simulink model "D53_LKAS_JLU_20200909_1512"  (R2018b)
settings: Solver=ode3  StartTime=0.0  StopTime=10.0  FixedStep=0.01  RelTol=1e-3  EnableMultiTasking=on
model workspace (MAT data in the model file):
  MCOS : class17 (value not decoded)
  MCOS : class17 (value not decoded)
  MCOS : class17 (value not decoded)
  MCOS : class17 (value not decoded)
  MCOS : class17 (value not decoded)
  MCOS : class17 (value not decoded)
  MCOS : class17 (value not decoded)
  MCOS : class17 (value not decoded)
  MCOS : class17 (value not decoded)
  MCOS : class17 (value not decoded)
  MCOS : class17 (value not decoded)
  MCOS : class17 (value not decoded)
  MCOS : class17 (value not decoded)
  MCOS : class17 (value not decoded)
  MCOS : class17 (value not decoded)
  MCOS : class17 (value not decoded)
  MCOS : class17 (value not decoded)
  MCOS : class17 (value not decoded)
  MCOS : class17 (value not decoded)
  MCOS : class17 (value not decoded)
  MCOS : class17 (value not decoded)
  MCOS : class17 (value not decoded)
  MCOS : class17 (value not decoded)
  MCOS : class17 (value not decoded)
  MCOS : class17 (value not decoded)
  MCOS : class17 (value not decoded)
  MCOS : class17 (value not decoded)
  MCOS : class17 (value not decoded)
  MCOS : class17 (value not decoded)
  MCOS : class17 (value not decoded)
  MCOS : class17 (value not decoded)
  MCOS : class17 (value not decoded)
  MCOS : class17 (value not decoded)
  MCOS : class17 (value not decoded)
  MCOS : class17 (value not decoded)
  MCOS : class17 (value not decoded)
  MCOS : class17 (value not decoded)
  MCOS : class17 (value not decoded)
  MCOS : class17 (value not decoded)
  MCOS : class17 (value not decoded)
  MCOS : class17 (value not decoded)
  MCOS : class17 (value not decoded)
  MCOS : class17 (value not decoded)
  MCOS : class17 (value not decoded)
  MCOS : class17 (value not decoded)
  MCOS : class17 (value not decoded)
  MCOS : class17 (value not decoded)
  MCOS : class17 (value not decoded)
  MCOS : class17 (value not decoded)
  MCOS : class17 (value not decoded)
  MCOS : class17 (value not decoded)
  MCOS : class17 (value not decoded)
  MCOS : class17 (value not decoded)
  MCOS : class17 (value not decoded)
  MCOS : class17 (value not decoded)
  MCOS : class17 (value not decoded)
  MCOS : class17 (value not decoded)
  MCOS : class17 (value not decoded)
  MCOS : class17 (value not decoded)
  MCOS : class17 (value not decoded)
  MCOS : class17 (value not decoded)
  MCOS : class17 (value not decoded)
  MCOS : class17 (value not decoded)
  MCOS : class17 (value not decoded)
  MCOS : class17 (value not decoded)
  MCOS : class17 (value not decoded)
  MCOS : class17 (value not decoded)
  MCOS : class17 (value not decoded)
  MCOS : class17 (value not decoded)
  MCOS : class17 (value not decoded)
  MCOS : class17 (value not decoded)
  MCOS : class17 (value not decoded)
  MCOS : class17 (value not decoded)
  MCOS : class17 (value not decoded)
  MCOS : class17 (value not decoded)
  MCOS : class17 (value not decoded)
  MCOS : class17 (value not decoded)
  MCOS : class17 (value not decoded)
  MCOS : class17 (value not decoded)
  MCOS : class17 (value not decoded)
  MCOS : class17 (value not decoded)
  MCOS : class17 (value not decoded)
  MCOS : class17 (value not decoded)
  MCOS : class17 (value not decoded)
  MCOS : class17 (value not decoded)
  MCOS : class17 (value not decoded)
  MCOS : class17 (value not decoded)
  MCOS : class17 (value not decoded)
  MCOS : class17 (value not decoded)
undefined symbols (not defined in the file): LKA_CarWidth, LKA_SampleTime, LKA_StrRatio_C, LKA_Veh2CamL_C, LKA_Veh2CamW_C, LKA_WhlBaseL_C, LL_CompSWA_C, LL_CrvtPrvwT_C, LL_DesDvt_C, LL_DvtComp_C, LL_DvtPrvwT_C, LL_DvtSpdDet_vDvtSpdMin_C, LL_HdAgExT_C, LL_HdAgPrvwT_C, LL_LAccMax_C, LL_LAccRMax_C, LL_LDW_EarliestWarnLine_C, LL_LDW_LatestWarnLine_C, LL_LDWS_SUPPRESS_HEADING, LL_LFClb_TFC_DiffCtlBalance, LL_LFClb_TFC_DiffCtrlMaxSWA, LL_LFClb_TFC_DiffCtrlRatio, LL_LFClb_TFC_facmGainLutGain1_C, LL_LFClb_TFC_facmGainLutGain2_C, LL_LFClb_TFC_facmIntegRatio, LL_LFClb_TFC_facmKlat_C, LL_LFClb_TFC_FfCtlRatio_C, LL_LFClb_TFC_phiIntegCtlMaxSWA_C, LL_LFClb_TFC_tiKlatPrvwT_C, LL_LFClb_TFC_vGainLutVehSpdLwr_C, LL_LFClb_TFC_vGainLutVehSpdUpr_C, LL_LKA_EarliestWarnLine_C, LL_LKA_LatestWarnLine_C, LL_LKAExPrcs_ExitC0Dvt, LL_LKAExPrcs_ExitC0Swt, LL_LKAExPrcs_tiExitTime1, LL_LKAExPrcs_tiExitTime2, LL_LKAExPrcs_tiExitTime3, LL_LKAS_OUT_OF_CONTROL_LAT_VEL, LL_LKAS_OUT_OF_CONTROL_TTLC, LL_LKASWASyn_M0, LL_LKASWASyn_M1, LL_LKASWASyn_M2, LL_LKASWASyn_M3K, LL_LKASWASyn_SWAaddMax, LL_LKASWASyn_T2, LL_LKASWASyn_tiTrqSwaRtTime, LL_LKASWASyn_tiTrqSwaTime, LL_LKASWASyn_TrqMax, LL_LKASWASyn_TrqSwaAddSwt, LL_LKASWASyn_TrqSwaRateDiff, LL_LSpdCompT_C, LL_lStpLngth_C, LL_MAX_DELAY_EPSSTAR_TIME, LL_MAX_DRIVER_TORQUE_DISABLE, LL_MAX_DRIVER_TORQUE_ENABLE, LL_MAX_LANE_WIDTH_DISABLE, LL_MAX_LANE_WIDTH_ENABLE, LL_MAX_LAT_ACC_DISABLE, LL_MAX_LAT_ACC_ENABLE ... (+30)
libraries: simulink x134, canmsglib x50, dspstat3 x3, simulink_extras x1
(part 9 of 17)

== system D53_LKAS_JLU_20200909_1512/LL/LLOn/LKA/Driver Torque Addition (DTA)/Subsystem ==
  DTA_bsInInfoSyn : Inport
  DTA_bsLFClb : Inport  Port=2
  LKA_SampleTime : Inport  Port=3
  Enable : EnablePort
  Add : Sum
  Bus Selector2 : BusSelector  OutputSignals=bsVehMovInfo.ESC_VehSpd,bsEPSInfo.EPS_SW_Trq,bsLaneInfo.bsL0Info.L0_C0,bsLaneInfo.bsR0Info.R0_C0
  Bus Selector4 : BusSelector  OutputSignals=LL_LKASWAClb.LL_LKASWASyn_SWAaddMax,LL_LKASWAClb.LL_LKASWASyn_TrqMax,LL_LKASWAClb.LL_LKASWASyn_TrqSwaAddSwt,LL_LKASWAClb.LL_LKASWASyn_tiTrqSwaTime,LL_LKASWAClb.LL_LKASWASyn_tiTrqSwaRtTime,LL_LKASWAClb.LL_LKASWASyn_TrqSwaRateDiff
  Constant1 : Constant  Value=5  OutDataTypeStr=single
  Constant2 : Constant  Value=-5  OutDataTypeStr=single
  Divide1 : Product  Inputs=***
  Divide3 : Product  Inputs=**
  DriverSwaTrqAdd : MATLAB Function  TreatAsAtomicUnit=on
  LowPass : Subsystem
  LowPass1 : Subsystem
  Rate Limiter Dynamic : simulink/Discontinuities/Rate Limiter Dynamic
      settings: SourceProductName=Simulink
  Saturation : Saturate  UpperLimit=30  LowerLimit=-30
  Out1 : Outport  OutputWhenDisabled=reset  InitialOutput=0
  wires:
  DTA_bsLFClb/1 -> Bus Selector4/1
  Bus Selector4/2 -> DriverSwaTrqAdd/6(trqmax)  "<LL_LKASWASyn_TrqMax>"
  LKA_SampleTime/1 -> LowPass1/3(dT), LowPass/3(dT)
  Bus Selector2/3 -> DriverSwaTrqAdd/3(l0c0)  "<L0_C0>"
  Bus Selector4/5 -> LowPass1/1(T)  "<LL_LKASWASyn_tiTrqSwaRtTime>"
  Bus Selector2/1 -> DriverSwaTrqAdd/1(spd)  "<ESC_VehSpd>"
  Bus Selector4/6 -> Divide1/3  "<LL_LKASWASyn_TrqSwaRateDiff>"
  Bus Selector2/4 -> DriverSwaTrqAdd/4(r0c0)  "<R0_C0>"
  Bus Selector2/2 -> DriverSwaTrqAdd/2(trq)  "<EPS_SW_Trq>"
  Divide1/1 -> Add/2  "SWARateAdd"
  LowPass/1(y) -> LowPass1/2(u), Divide3/2  "TrqSWAAdd"
  Bus Selector4/4 -> LowPass/1(T)  "<LL_LKASWASyn_tiTrqSwaTime>"
  DTA_bsInInfoSyn/1 -> Bus Selector2/1
  Saturation/1 -> Divide1/2
  Rate Limiter Dynamic/1 -> Out1/1
  DriverSwaTrqAdd/1(Swaadd) -> LowPass/2(u)  "TrqSWAAddRaw"
  Constant1/1 -> Rate Limiter Dynamic/1
  Bus Selector4/1 -> DriverSwaTrqAdd/5(swaaddmax)  "<LL_LKASWASyn_SWAaddMax>"
  Constant2/1 -> Rate Limiter Dynamic/3
  Divide3/1 -> Add/1  "TrqSWAAdd"
  LowPass1/1(y) -> Saturation/1  "SWARateAdd"
  Bus Selector4/3 -> Divide1/1, Divide3/1  "<LL_LKASWASyn_TrqSwaAddSwt>"
  Add/1 -> Rate Limiter Dynamic/2

== system D53_LKAS_JLU_20200909_1512/LL/LLOn/LKA/Driver Torque Addition (DTA)/Subsystem1 ==
  DTA_bsInInfoSyn : Inport
  DTA_bsLFClb : Inport  Port=2
  Add1 : Sum  Inputs=-+
  Bus Selector : BusSelector  OutputSignals=bsEPSInfo.EPS_SW_Trq
  Bus Selector1 : BusSelector  OutputSignals=LL_LKASWAClb.LL_LKASWASyn_M3K,LL_LKASWAClb.LL_LKASWASyn_M0,LL_LKASWAClb.LL_LKASWASyn_M1,LL_LKASWAClb.LL_LKASWASyn_M2,LL_LKASWAClb.LL_LKASWASyn_T2
  Divide : Product  Inputs=**
  MATLAB Function : MATLAB Function  TreatAsAtomicUnit=on
  Moving Standard Deviation2 : Subsystem  TreatAsAtomicUnit=on
      mask Display: disp(['Moving' char(10) 'Standard' char(10) 'Deviation']);
  Saturation1 : Saturate  UpperLimit=0.2  LowerLimit=0
  Saturation2 : Saturate  UpperLimit=1  LowerLimit=0
  TickTime (TTime) : Subsystem
      mask Display:
      | port_label('output', 1, 'TTime');
      | color('blue');
      | text(0.98,0.9,'VCDC Block','horizontalAlignment','right');
      | color('black');
      | text(0.5,0.55,'Tick Time','horizontalAlignment','center');
      | text(0.5,0.4,'(TTime)','horizontalAlignment','center');
  Out1 : Outport
  wires:
  Saturation2/1 -> Out1/1
  DTA_bsLFClb/1 -> Bus Selector1/1
  DTA_bsInInfoSyn/1 -> Bus Selector/1
  Moving Standard Deviation2/1(Out1) -> Divide/1
  Bus Selector/1 -> Moving Standard Deviation2/1(In1)  "<EPS_SW_Trq>"
  Bus Selector1/4 -> MATLAB Function/3(M2)  "<LL_LKASWASyn_M2>"
  Bus Selector1/1 -> Divide/2  "<LL_LKASWASyn_M3K>"
  Add1/1 -> Saturation2/1
  Divide/1 -> Saturation1/1
  TickTime (TTime)/1(Out1) -> [T]
  Bus Selector1/5 -> MATLAB Function/5(T2)  "<LL_LKASWASyn_T2>"
  MATLAB Function/1(M) -> Add1/2
  Saturation1/1 -> Add1/1  "M3"
  [T] -> MATLAB Function/6(T)
  [PT1] -> MATLAB Function/4(T1)
  Bus Selector1/3 -> MATLAB Function/2(M1)  "<LL_LKASWASyn_M1>"
  Bus Selector1/2 -> MATLAB Function/1(M0)  "<LL_LKASWASyn_M0>"

== system D53_LKAS_JLU_20200909_1512/LL/LLOn/LKA/LKA Exit Processing (LKAExPrcs)/Exit Time 1 ==
  bsLKAInPInfo : Inport
  bsLKAClb : Inport  Port=2
  Abs : Abs
  Add : Sum
  Add2 : Sum  OutDataTypeStr=single
  Bus Selector1 : BusSelector  OutputSignals=LL_LKAExPrcs.LL_LKAExPrcs_tiExitTime1
  Bus Selector2 : BusSelector  OutputSignals=Pr_bsPrInfo.bsPrCrvtInfo.crPrvwCrvt
  Constant : Constant  Value=0.004  OutDataTypeStr=single
  Constant1 : Constant  Value=0.5  OutDataTypeStr=single
  Divide : Product  Inputs=***/
  Memory : Memory  InheritSampleTime=on
  Relational Operator4 : RelationalOperator  OutDataTypeStr=boolean  RndMeth=Nearest
  Saturation : Saturate  UpperLimit=0.004  LowerLimit=0
  Saturation2 : Saturate  UpperLimit=10  LowerLimit=0
  Exit1 : Outport
  wires:
  Bus Selector1/1 -> Divide/1, Add/1  "<LL_LKAExPrcs_tiExitTime1>"
  Saturation/1 -> Divide/3
  Add/1 -> Relational Operator4/2
  Abs/1 -> Saturation/1
  Divide/1 -> Add/2
  Bus Selector2/1 -> Abs/1  "<crPrvwCrvt>"
  Constant1/1 -> Divide/2
  Constant/1 -> Divide/4
  bsLKAInPInfo/1 -> Bus Selector2/1
  Relational Operator4/1 -> Exit1/1
  Memory/1 -> Add2/2
  Saturation2/1 -> Memory/1
  bsLKAClb/1 -> Bus Selector1/1
  Add2/1 -> Relational Operator4/1, Saturation2/1
  [LKA_SampleTime] -> Add2/1

== system D53_LKAS_JLU_20200909_1512/LL/LLOn/LKA/LKA Exit Processing (LKAExPrcs)/Exit Time 2 ==
  bsInInfoSyn : Inport
  bsLKAClb : Inport  Port=2
  bsLKAInPInfo : Inport  Port=3
  T1 : Inport  Port=4
  Abs : Abs
  Abs2 : Abs
  Abs3 : Abs
  Add : Sum
  Add1 : Sum
  Add2 : Sum  OutDataTypeStr=single
  Bus Selector : BusSelector  OutputSignals=LKA_Veh2CamW_C
  Bus Selector1 : BusSelector  OutputSignals=Pr_bsPrInfo.bsPrCrvtInfo.crPrvwCrvt
  Bus Selector2 : BusSelector  OutputSignals=bsLaneInfo.bsL0Info.L0_C0,bsLaneInfo.bsR0Info.R0_C0
  Bus Selector3 : BusSelector  OutputSignals=LL_LKAExPrcs.LL_LKAExPrcs_tiExitTime2
  Constant : Constant  Value=0.004  OutDataTypeStr=single
  Constant1 : Constant  Value=0.5  OutDataTypeStr=single
  Constant3 : Constant  Value=0.3  OutDataTypeStr=single
  Divide : Product  Inputs=***/
  Logical Operator1 : Logic  Inputs=3  AllPortsSameDT=off  OutDataTypeStr=boolean
  Memory : Memory  InheritSampleTime=on
  Relational Operator2 : RelationalOperator  OutDataTypeStr=boolean  RndMeth=Nearest
  Relational Operator3 : RelationalOperator  OutDataTypeStr=boolean  RndMeth=Nearest
  Relational Operator4 : RelationalOperator  OutDataTypeStr=boolean  RndMeth=Nearest
  Saturation : Saturate  UpperLimit=0.004  LowerLimit=0
  Saturation2 : Saturate  UpperLimit=10  LowerLimit=0
  Sum Condition1 : Subsystem
  Exit2 : Outport
  wires:
  bsLKAClb/1 -> Bus Selector3/1
  [LKA_ConstantClb] -> Bus Selector/1
  Bus Selector/1 -> Add/2  "<LKA_Veh2CamW_C>"
  Saturation/1 -> Divide/3
  Bus Selector3/1 -> Add1/1, Divide/1  "<LL_LKAExPrcs_tiExitTime2>"
  Divide/1 -> Add1/2
  Constant1/1 -> Divide/2
  Abs/1 -> Saturation/1
  Constant/1 -> Divide/4
  Add1/1 -> Sum Condition1/2(Time Exit 2)
  Bus Selector1/1 -> Abs/1  "<crPrvwCrvt>"
  bsLKAInPInfo/1 -> Bus Selector1/1
  bsInInfoSyn/1 -> Bus Selector2/1
  [LKA_SampleTime] -> Sum Condition1/1(Sample Time)
  Sum Condition1/1(Out) -> Exit2/1
  T1/1 -> Relational Operator4/2
  [LKA_SampleTime] -> Add2/1
  Memory/1 -> Add2/2
  Add2/1 -> Relational Operator4/1, Saturation2/1
  Relational Operator4/1 -> Logical Operator1/1
  Saturation2/1 -> Memory/1
  Constant3/1 -> Add/1
  Logical Operator1/1 -> Sum Condition1/Enable
  Relational Operator3/1 -> Logical Operator1/3
  Abs2/1 -> Relational Operator2/1
  Bus Selector2/1 -> Abs2/1  "<L0_C0>"
  Relational Operator2/1 -> Logical Operator1/2
  Abs3/1 -> Relational Operator3/1
  Bus Selector2/2 -> Abs3/1  "<R0_C0>"
  Add/1 -> Relational Operator2/2, Relational Operator3/2

== system D53_LKAS_JLU_20200909_1512/LL/LLOn/LKA/LKA Exit Processing (LKAExPrcs)/Exit Time 3 ==
  bsInInfoSyn : Inport
  bsLKAInPInfo : Inport  Port=2
  bsLKAClb : Inport  Port=3
  T1 : Inport  Port=4
  Abs2 : Abs
  Abs3 : Abs
  Abs4 : Abs
  Add : Sum
  Add2 : Sum  OutDataTypeStr=single
  Add4 : Sum
  Add5 : Sum  Inputs=+-
  Add6 : Sum
  Bus Selector : BusSelector  OutputSignals=LKA_Veh2CamW_C
  Bus Selector1 : BusSelector  OutputSignals=bsLaneInfo.bsL0Info.L0_C0,bsLaneInfo.bsR0Info.R0_C0
  Bus Selector2 : BusSelector  OutputSignals=bsLaneInfo.bsL0Info.L0_C0,bsLaneInfo.bsR0Info.R0_C0
  Bus Selector3 : BusSelector  OutputSignals=LL_LKAExPrcs.LL_LKAExPrcs_tiExitTime3,LL_LKAExPrcs.LL_LKAExPrcs_ExitC0Dvt,LL_LKAExPrcs.LL_LKAExPrcs_ExitC0Swt
  Bus Selector4 : BusSelector  OutputSignals=Pr_bsPrInfo.bsPrCrvtInfo.crPrvwCrvt
  Constant : Constant  Value=0.004  OutDataTypeStr=single
  Constant4 : Constant  Value=0.3  OutDataTypeStr=single
  Constant7 : Constant  Value=2  OutDataTypeStr=single
  Divide1 : Product  Inputs=**/
  Divide2 : Product  Inputs=*/
  Gain : Gain  Gain=0.25
  Logical Operator1 : Logic  Inputs=3  AllPortsSameDT=off  OutDataTypeStr=boolean
  Logical Operator2 : Logic  Inputs=4  AllPortsSameDT=off  OutDataTypeStr=boolean
  Memory : Memory  InheritSampleTime=on
  Moving Standard Deviation1 : Subsystem  TreatAsAtomicUnit=on
      mask Display: disp(['Moving' char(10) 'Standard' char(10) 'Deviation']);
  Moving Standard Deviation2 : Subsystem  TreatAsAtomicUnit=on
      mask Display: disp(['Moving' char(10) 'Standard' char(10) 'Deviation']);
  Relational Operator2 : RelationalOperator  OutDataTypeStr=boolean  RndMeth=Nearest
  Relational Operator3 : RelationalOperator  OutDataTypeStr=boolean  RndMeth=Nearest
  Relational Operator4 : RelationalOperator  OutDataTypeStr=boolean  RndMeth=Nearest
  Relational Operator5 : RelationalOperator  Operator=<=  OutDataTypeStr=boolean  RndMeth=Nearest
  Relational Operator6 : RelationalOperator  Operator=<=  OutDataTypeStr=boolean  RndMeth=Nearest
  Saturation : Saturate  UpperLimit=0.004  LowerLimit=0
  Saturation1 : Saturate  UpperLimit=5.5  LowerLimit=2.4
  Saturation2 : Saturate  UpperLimit=10  LowerLimit=0
  Sum Condition : Subsystem
  Sum Condition1 : Subsystem
  Exit3 : Outport
  wires:
  Add6/1 -> Divide2/1
  [LKA_SampleTime] -> Divide2/2
  Constant7/1 -> Divide1/1
  Bus Selector4/1 -> Abs4/1  "<crPrvwCrvt>"
  Saturation/1 -> Divide1/2
  Abs4/1 -> Saturation/1
  Divide1/1 -> Add6/2
  Constant/1 -> Divide1/3
  bsLKAInPInfo/1 -> Bus Selector4/1
  Moving Standard Deviation1/1(Out1) -> Relational Operator6/1
  Divide2/1 -> Sum Condition1/2(In1), Sum Condition/2(In1)
  Relational Operator6/1 -> Sum Condition1/1(In), Sum Condition1/Enable
  Sum Condition1/1(Out) -> Logical Operator2/2
  Sum Condition/1(Out) -> Logical Operator2/3
  Relational Operator5/1 -> Sum Condition/1(In), Sum Condition/Enable
  Gain/1 -> Add5/1
  Constant4/1 -> Add5/2
  Saturation1/1 -> Gain/1
  Add4/1 -> Saturation1/1
  Moving Standard Deviation2/1(Out1) -> Relational Operator5/1
  [LKA_ConstantClb] -> Bus Selector/1
  Bus Selector/1 -> Add/2  "<LKA_Veh2CamW_C>"
  Logical Operator2/1 -> Exit3/1
  Bus Selector1/1 -> Moving Standard Deviation2/1(In1)  "<L0_C0>"
  Bus Selector1/2 -> Moving Standard Deviation1/1(In1)  "<R0_C0>"
  bsLKAClb/1 -> Bus Selector3/1
  Bus Selector3/2 -> Relational Operator6/2, Relational Operator5/2  "<LL_LKAExPrcs_ExitC0Dvt>"
  bsInInfoSyn/1 -> Bus Selector1/1, Bus Selector2/1
  Bus Selector3/3 -> Logical Operator2/4  "<LL_LKAExPrcs_ExitC0Swt>"
  Bus Selector3/1 -> Add6/1  "<LL_LKAExPrcs_tiExitTime3>"
  Add/1 -> Relational Operator3/2, Relational Operator2/2
  Bus Selector2/2 -> Abs3/1  "<R0_C0>"
  Abs3/1 -> Relational Operator3/1, Add4/2
  Relational Operator2/1 -> Logical Operator1/2
  Bus Selector2/1 -> Abs2/1  "<L0_C0>"
  Abs2/1 -> Add4/1, Relational Operator2/1
  Relational Operator3/1 -> Logical Operator1/3
  Logical Operator1/1 -> Logical Operator2/1
  Add5/1 -> Add/1
  Saturation2/1 -> Memory/1
  Relational Operator4/1 -> Logical Operator1/1
  Add2/1 -> Saturation2/1, Relational Operator4/1
  Memory/1 -> Add2/2
  [LKA_SampleTime] -> Add2/1
  T1/1 -> Relational Operator4/2

== system D53_LKAS_JLU_20200909_1512/LL/LLOn/LKA/LKA Motion Planning (LKAMP) /LKA Motion Planning Calculation (LKAMPCal) ==
  LKAMPCal_bsLKAInPInfo : Inport
  LKAMPCal_bsLKAClb : Inport  Port=2
  LLClb_bsConstantClb : Inport  Port=3
  Action Port : ActionPort  InitializeStates=reset  ActionType=then
  Bus Creator : BusCreator  Inputs=6
  Bus Creator3 : BusCreator  Inputs=5
  Bus Creator5 : BusCreator  Inputs=3
  Bus Selector : BusSelector  OutputSignals=MPInP_stLDDir,MPInP_tiTTLCIni,MPInP_vVehSpdIni,MPInP_phiSWAIni,MPInP_phiPrvwHdAgIni,MPInP_phiHdAgIni,MPInP_phiHdAgMax,MPInP_lDvtIni,UndrLim_dphiSWARMax,StbFacm_SY
  Bus Selector1 : BusSelector  OutputSignals=LL_DesDvt_C,LL_lStpLngth_C
  Bus Selector2 : BusSelector  OutputSignals=LKA_WhlBaseL_C,LKA_StrRatio_C
  Bus Selector3 : BusSelector  OutputSignals=signal1,signal2,signal3,signal4,signal5
  Bus Selector4 : BusSelector  OutputSignals=LKA_WhlBaseL_C,LKA_StrRatio_C,StbFacm_SY
  MATLAB Function : MATLAB Function  TreatAsAtomicUnit=on
  Memory{,1..4} (5 alike) : Memory  InheritSampleTime=on
  Time Division (TDiv) : Subsystem
  Time Division (TDiv)1 : Subsystem
  Time Division (TDiv)2 : Subsystem
  Time Division (TDiv)3 : Subsystem
  Time Division (TDiv)4 : Subsystem
  LKAMPCal_bsLKAMPCalOut : Outport
  wires:
  LKAMPCal_bsLKAInPInfo/1 -> Bus Selector/1
  LKAMPCal_bsLKAClb/1 -> Bus Selector1/1
  Bus Creator/1 -> LKAMPCal_bsLKAMPCalOut/1  "LKAMPCal_bsLKAMPCalOut"
  MATLAB Function/2(K1K2Det_dphi2PhSWAGrad1) -> Bus Creator/2
  MATLAB Function/5(K1K2Det_stReplFlag) -> Bus Creator/5
  MATLAB Function/3(K1K2Det_dphi2PhSWAGrad2) -> Bus Creator/3
  MATLAB Function/1(K1K2Det_dphi1PhSWAGrad) -> Bus Creator/1
  Bus Selector/3 -> MATLAB Function/3(K1K2Det_vVehSpd)  "<MPInP_vVehSpdIni>"
  Bus Selector/7 -> MATLAB Function/8(K1K2Det_phi2PhDesHdAg)  "<MPInP_phiHdAgMax>"
  Bus Selector/1 -> MATLAB Function/1(K1K2Det_stLDDir)  "<MPInP_stLDDir>"
  Bus Selector2/1 -> Bus Creator5/1  "<LKA_WhlBaseL_C>"
  Bus Selector2/2 -> Bus Creator5/2  "<LKA_StrRatio_C>"
  Bus Selector/10 -> Bus Creator5/3  "<StbFacm_SY>"
  Bus Selector1/1 -> MATLAB Function/17(K1K2Det_lDesDvt)  "<LL_DesDvt_C>"
  Bus Selector/8 -> MATLAB Function/9(K1K2Det_l1PhDvtIni)  "<MPInP_lDvtIni>"
  Bus Selector1/2 -> MATLAB Function/18(K1K2Det_lStpLngth)  "<LL_lStpLngth_C>"
  Bus Selector/4 -> MATLAB Function/4(K1K2Det_phiIniSWA)  "<MPInP_phiSWAIni>"
  MATLAB Function/4(K1K2Det_phi2PhSWAIni) -> Bus Creator/4  "K1K2Det_phi2PhSWAIni"
  Bus Selector/2 -> MATLAB Function/2(K1K2Det_tiTTLC0)  "<MPInP_tiTTLCIni>"
  Bus Selector/6 -> MATLAB Function/7(K1K2Det_phi1PhDesHdAgIni)  "<MPInP_phiHdAgIni>"
  Bus Selector/5 -> MATLAB Function/5(K1K2Det_phiPrvwHdAgIni)  "<MPInP_phiPrvwHdAgIni>"
  MATLAB Function/6(K1K2Det_dphi1PhHdAgIni) -> Bus Creator/6
  Bus Selector/9 -> MATLAB Function/10(K1K2Det_dphiSWARMax)  "<UndrLim_dphiSWARMax>"
  LLClb_bsConstantClb/1 -> Bus Selector2/1
  Bus Selector3/4 -> MATLAB Function/15(K1K2Det_bsTDivInfo_Ph2DvtEnd)  "<signal4>"
  Bus Selector3/3 -> MATLAB Function/14(K1K2Det_bsTDivInfo_Mode2Num)  "<signal3>"
  Bus Selector3/1 -> MATLAB Function/12(K1K2Det_bsTDivInfo_ModeFlg)  "<signal1>"
  Bus Selector3/2 -> MATLAB Function/13(K1K2Det_bsTDivInfo_Mode1Num)  "<signal2>"
  Bus Selector3/5 -> MATLAB Function/16(K1K2Det_bsTDivInfo_Ph2SWAIni)  "<signal5>"
  Bus Selector4/1 -> MATLAB Function/19(K1K2Det_bsSysCfg_SY_WhlBase_SY)  "<LKA_WhlBaseL_C>"
  Bus Selector4/3 -> MATLAB Function/21(K1K2Det_bsSysCfg_SY_StbFacm_SY)  "<StbFacm_SY>"
  Bus Selector4/2 -> MATLAB Function/20(K1K2Det_bsSysCfg_SY_StRatio_SY)  "<LKA_StrRatio_C>"
  Bus Creator5/1 -> Bus Selector4/1
  MATLAB Function/7(K1K2Det_bsTDivInfoOut_ModeFlg) -> Memory/1
  Memory/1 -> Time Division (TDiv)/1(TDiv_bsTDivInfoOut)
  Bus Creator3/1 -> Bus Selector3/1
  Memory1/1 -> Time Division (TDiv)1/1(TDiv_bsTDivInfoOut1)
  MATLAB Function/8(K1K2Det_bsTDivInfoOut_Mode1Num) -> Memory1/1
  MATLAB Function/9(K1K2Det_bsTDivInfoOut_Mode2Num) -> Memory2/1
  Memory2/1 -> Time Division (TDiv)2/1(TDiv_bsTDivInfoOut1)
  Memory3/1 -> Time Division (TDiv)3/1(TDiv_bsTDivInfoOut1)
  MATLAB Function/10(K1K2Det_bsTDivInfoOut_Ph2DvtEnd) -> Memory3/1
  MATLAB Function/11(K1K2Det_bsTDivInfoOut_Ph2SWAIni) -> Memory4/1
  Memory4/1 -> Time Division (TDiv)4/1(TDiv_bsTDivInfoOut1)
  Time Division (TDiv)/1(Out1) -> Bus Creator3/1
  Time Division (TDiv)1/1(Out2) -> Bus Creator3/2
  Time Division (TDiv)2/1(Out2) -> Bus Creator3/3
  Time Division (TDiv)3/1(Out2) -> Bus Creator3/4
  Time Division (TDiv)4/1(Out2) -> Bus Creator3/5

== system D53_LKAS_JLU_20200909_1512/LL/LLOn/LKA/LKA Motion Planning (LKAMP) /Motion Planning Input Processing (MPInP) ==
  MPInP_stLKAActvFlg : Inport
  MPInP_phiHdAgMax : Inport  Port=2
  MPInP_bsLKAInPInfo : Inport  Port=3
  MPInP_bsInInfoSyn : Inport  Port=4
  Bus Creator : BusCreator  Inputs=11
  Bus Selector1 : BusSelector  OutputSignals=TTLC_bsTTLCInfo.LFTTTLC,TTLC_bsTTLCInfo.RGTTTLC
  Bus Selector3 : BusSelector  OutputSignals=bsSWAInfo.SW_Angle,bsVehMovInfo.ESC_VehSpd
  Bus Selector4 : BusSelector  OutputSignals=Pr_bsPrInfo.bsPrHdAgInfo.phiPrvwTTLCHdAg,Pr_bsPrInfo.bsPrDvtInfo.lDvt,Pr_bsPrInfo.bsPrHdAgInfo.phiHdAg,UndrLim_dphiSWARMax
  Cast To Single1 : DataTypeConversion  LockScale=on
  Lane Information Selection (LaneInfoSel) : Subsystem
  Lookup Table2 : Lookup_n-D  NumberOfTableDimensions=1  BreakpointsForDimension1=[11.7,18.83,26.98,31.98,51.04,79,86.08,90.59]  BeginIndexSearchUsingPreviousIndexResult=on  Table=[0.012141,0.005179,0.00298,0.002547,0.001715,0.001283,0.001021,0.000982]  RemoveProtectionInput=on  InternalRulePriority=Speed  OutDataTypeStr=single  InputSameDT=on
  MATLAB Function : MATLAB Function  TreatAsAtomicUnit=on
  Saturation : Saturate  UpperLimit=20  LowerLimit=-20
  Saturation1 : Saturate  UpperLimit=0.0117  LowerLimit=0.00237
  Saturation2 : Saturate  UpperLimit=2  LowerLimit=0.6
  Signal Latching2 : Subsystem  mask(Signal Latching:){LatchTime=1}
      mask prompts: LatchTime "Latch time(-):"
      mask help:
      | If the latch time is not reached, the input signal will just go through the block. If the latch time is reached, the output will be held and do not change again. The latch time is described with the number of the sampling time.
      | ----vcdc.ascl@jlu 19-01-15
  Signal Latching3 : Subsystem  mask(Signal Latching:){LatchTime=1}
      mask prompts: LatchTime "Latch time(-):"
      mask help:
      | If the latch time is not reached, the input signal will just go through the block. If the latch time is reached, the output will be held and do not change again. The latch time is described with the number of the sampling time.
      | ----vcdc.ascl@jlu 19-01-15
  Signal Latching4 : Subsystem  mask(Signal Latching:){LatchTime=1}
      mask prompts: LatchTime "Latch time(-):"
      mask help:
      | If the latch time is not reached, the input signal will just go through the block. If the latch time is reached, the output will be held and do not change again. The latch time is described with the number of the sampling time.
      | ----vcdc.ascl@jlu 19-01-15
  Signal Latching5 : Subsystem  mask(Signal Latching:){LatchTime=1}
      mask prompts: LatchTime "Latch time(-):"
      mask help:
      | If the latch time is not reached, the input signal will just go through the block. If the latch time is reached, the output will be held and do not change again. The latch time is described with the number of the sampling time.
      | ----vcdc.ascl@jlu 19-01-15
  Signal Latching6 : Subsystem  mask(Signal Latching:){LatchTime=1}
      mask prompts: LatchTime "Latch time(-):"
      mask help:
      | If the latch time is not reached, the input signal will just go through the block. If the latch time is reached, the output will be held and do not change again. The latch time is described with the number of the sampling time.
      | ----vcdc.ascl@jlu 19-01-15
  Signal Latching7 : Subsystem  mask(Signal Latching:){LatchTime=1}
      mask prompts: LatchTime "Latch time(-):"
      mask help:
      | If the latch time is not reached, the input signal will just go through the block. If the latch time is reached, the output will be held and do not change again. The latch time is described with the number of the sampling time.
      | ----vcdc.ascl@jlu 19-01-15
  Subsystem : Subsystem
  MPInP_bsMPInPInfo : Outport
  wires:
  Saturation2/1 -> Bus Creator/2  "MPInP_tiTTLCIni"
  Bus Creator/1 -> MPInP_bsMPInPInfo/1
  Lookup Table2/1 -> Saturation1/1
  Subsystem/1(Out6) -> Bus Creator/1  "MPInP_stLDDir"
  MPInP_bsInInfoSyn/1 -> Bus Selector3/1
  Bus Selector3/2 -> Lookup Table2/1, Cast To Single1/1, Signal Latching7/1(In)  "<ESC_VehSpd>"
  Signal Latching7/1(Out) -> Bus Creator/9  "MPInP_vVehSpdIni"
  Signal Latching5/1(Out) -> Saturation2/1  "MPInP_tiTTLCIni"
  Saturation1/1 -> Bus Creator/11  "StbFacm_SY"
  MPInP_stLKAActvFlg/1 -> Lane Information Selection (LaneInfoSel)/1(LaneInfoSel_stLKAActvFlg), Subsystem/1(In1)
  Signal Latching3/1(Out) -> Bus Creator/4  "MPInP_lDvtIni"
  Signal Latching2/1(Out) -> Bus Creator/3  "MPInP_phiPrvwHdAgIni"
  Signal Latching4/1(Out) -> Bus Creator/5  "MPInP_phiHdAgIni"
  Bus Selector4/2 -> Signal Latching3/1(In)  "<lDvt>"
  MPInP_phiHdAgMax/1 -> Bus Creator/7  "MPInP_phiHdAgMax"
  Bus Selector3/1 -> MATLAB Function/2(phiSWA), Signal Latching6/1(In)  "<SW_Angle>"
  Bus Selector4/3 -> Signal Latching4/1(In)  "<phiHdAg>"
  Cast To Single1/1 -> Bus Creator/10  "MPInP_vVehSpd"
  MPInP_bsLKAInPInfo/1 -> Bus Selector4/1, Bus Selector1/1
  Lane Information Selection (LaneInfoSel)/1(LaneInfoSel_facmActvLane) -> Signal Latching5/1(In)
  Bus Selector1/1 -> Lane Information Selection (LaneInfoSel)/2(LaneInfoSel_facmLftLane)  "<LFTTTLC>"
  Bus Selector1/2 -> Lane Information Selection (LaneInfoSel)/3(LaneInfoSel_facmRgtLane)  "<RGTTTLC>"
  Bus Selector4/4 -> Bus Creator/6  "<UndrLim_dphiSWARMax>"
  Bus Selector4/1 -> Signal Latching2/1(In)  "<phiPrvwTTLCHdAg>"
  Signal Latching6/1(Out) -> Bus Creator/8  "MPInP_phiSWAIni"
  [ActFlg] -> MATLAB Function/1(Actflg)
  [Ff] -> Saturation/1
  Saturation/1 -> MATLAB Function/3(phiFf)

== system D53_LKAS_JLU_20200909_1512/LL/LLOn/LKA/LKA Motion Planning (LKAMP) /Nominal Time Calculation (NomTCalc) ==
  NomTCalc_vVehSpd : Inport
  NomTCalc_vVehSpdIni : Inport  Port=2
  Add : Sum  OutDataTypeStr=single
  Divide : Product  Inputs=*/  OutDataTypeStr=single
  Gain : Gain  Gain=1/3.6  OutDataTypeStr=single
  Gain1 : Gain  Gain=1/3.6  OutDataTypeStr=single
  Memory : Memory  InheritSampleTime=on
  Product : Product
  NomTCalc_tiNomT : Outport
  wires:
  NomTCalc_vVehSpd/1 -> Gain/1
  Add/1 -> NomTCalc_tiNomT/1, Memory/1
  Memory/1 -> Add/2
  Gain/1 -> Product/1
  NomTCalc_vVehSpdIni/1 -> Gain1/1
  Gain1/1 -> Divide/2
  Product/1 -> Divide/1
  Divide/1 -> Add/1
  [LKA_SampleTime] -> Product/2

== system D53_LKAS_JLU_20200909_1512/LL/LLOn/LKA/LKA Motion Planning (LKAMP) /Steering Wheel Angle Command Calculation (SWACmdCal) ==
  SWACmdCal_bsK1K2DetOut : Inport
  SWACmdCal_bsLKAInPInfo : Inport  Port=2
  SWACmdCal_tiNomT : Inport  Port=3
  Bus Selector : BusSelector  OutputSignals=K1K2Det_dphi1PhSWAGrad,K1K2Det_phi2PhSWAIni,K1K2Det_dphi2PhSWAGrad1
  Bus Selector1 : BusSelector  OutputSignals=MPInP_phiSWAIni
  SWACmd : MATLAB Function  TreatAsAtomicUnit=on
  SWACmdCal_phiSWACmd : Outport
  SWACmdCal_tiT1 : Outport  Port=2
  SWACmdCal_tiT2 : Outport  Port=3
  wires:
  SWACmd/2(T1) -> SWACmdCal_tiT1/1
  SWACmdCal_tiNomT/1 -> SWACmd/5(SWACmd_tiNomT)
  Bus Selector1/1 -> SWACmd/4(SWACmd_phi1PhSWAIni)  "<MPInP_phiSWAIni>"
  SWACmdCal_bsLKAInPInfo/1 -> Bus Selector1/1
  Bus Selector/1 -> SWACmd/1(SWACmd_dphi1PhSWAGrad)  "<K1K2Det_dphi1PhSWAGrad>"
  Bus Selector/3 -> SWACmd/3(SWACmd_dphi2PhSWAGrad)  "<K1K2Det_dphi2PhSWAGrad1>"
  Bus Selector/2 -> SWACmd/2(SWACmd_phi2PhSWAIni)  "<K1K2Det_phi2PhSWAIni>"
  SWACmdCal_bsK1K2DetOut/1 -> Bus Selector/1
  SWACmd/1(SWACmd_phiSWACmd) -> SWACmdCal_phiSWACmd/1
  SWACmd/3(T2) -> SWACmdCal_tiT2/1

== system D53_LKAS_JLU_20200909_1512/LL/LLOn/LKA/LKA Motion Planning (LKAMP) /Switching Condition (SwtCon) ==
  SwtCon_stLKAActvFlg : Inport
  SwtCon_bsLKAInPInfo : Inport  Port=2
  SwtCon_vVehSpd : Inport  Port=3
  SwtCon_lLaneWidth_C : Inport  Port=4
  SwtCon_lCarWidth_C : Inport  Port=5
  SwtCon_tiHdAgExTime_C : Inport  Port=6
  SwtCon_tiLSpdCompT_C : Inport  Port=7
  Bus Selector1 : BusSelector  OutputSignals=Pr_bsPrInfo.bsPrCrvtInfo.crPrvwCrvt
  Ending Heading Angle Determination (EndHdAgDet) : Subsystem
  If : If  IfExpression=u1==1  ElseIfExpressions=u1==2
  If Action Subsystem : Subsystem  TreatAsAtomicUnit=on
  If Action Subsystem1 : Subsystem  TreatAsAtomicUnit=on
  If Action Subsystem2 : Subsystem  TreatAsAtomicUnit=on
  Merge : Merge  Inputs=3
  Signal Latching : Subsystem  mask(Signal Latching:){LatchTime=1}
      mask prompts: LatchTime "Latch time(-):"
      mask help:
      | If the latch time is not reached, the input signal will just go through the block. If the latch time is reached, the output will be held and do not change again. The latch time is described with the number of the sampling time.
      | ----vcdc.ascl@jlu 19-01-15
  SwtCon_phiHdAgMax : Outport
  wires:
  If/1 -> If Action Subsystem/Action
  If Action Subsystem/1(Out1) -> Merge/1
  If/2 -> If Action Subsystem1/Action
  If Action Subsystem1/1(Out1) -> Merge/2
  If/3 -> If Action Subsystem2/Action
  If Action Subsystem2/1(Out1) -> Merge/3
  SwtCon_lLaneWidth_C/1 -> Ending Heading Angle Determination (EndHdAgDet)/4(EndHdAgDet_lLaneWidth_C)
  SwtCon_lCarWidth_C/1 -> Ending Heading Angle Determination (EndHdAgDet)/5(EndHdAgDet_lCarWidth_C)
  SwtCon_tiHdAgExTime_C/1 -> Ending Heading Angle Determination (EndHdAgDet)/6(EndHdAgDet_tiHdAgExTime_C)
  SwtCon_vVehSpd/1 -> Ending Heading Angle Determination (EndHdAgDet)/2(EndHdAgDet_vVehSpd)
  Ending Heading Angle Determination (EndHdAgDet)/1(EndHdAgDet_phiHdAgMax) -> If Action Subsystem1/1(In1), If Action Subsystem/1(In1)
  Merge/1 -> Signal Latching/1(In)
  SwtCon_stLKAActvFlg/1 -> If/1, Ending Heading Angle Determination (EndHdAgDet)/1(EndHdAgDet_stLKAActvFlg)
  Signal Latching/1(Out) -> SwtCon_phiHdAgMax/1
  SwtCon_tiLSpdCompT_C/1 -> Ending Heading Angle Determination (EndHdAgDet)/7(EndHdAgDet_tiLSpdCompT_C)
  SwtCon_bsLKAInPInfo/1 -> Bus Selector1/1
  Bus Selector1/1 -> Ending Heading Angle Determination (EndHdAgDet)/3(EndHdAgDet_crPrvwCrvt)  "<crPrvwCrvt>"

== system D53_LKAS_JLU_20200909_1512/LL/LLOn/LKA/LKA SWA Limit (LKASWALim)/Rate Limiter Dynamic  ==
  note: U(k)
  note: Y(k)
  up : Inport
  u : Inport  Port=2
  lo : Inport  Port=3
  Add1 : Sum  OutDataTypeStr=uint16
  Constant : Constant  OutDataTypeStr=uint16  SampleTime=-1
  Delay Input2 : UnitDelay  Description=Store in Global RAM  DisableCoverage=on  SampleTime=-1
  Difference Inputs1 : Sum  Description=Add in CPU  DisableCoverage=on  Inputs=+-  OutDataTypeStr=Inherit: Inherit via back propagation
  Difference Inputs2 : Sum  Description=Add in CPU  OutDataTypeStr=Inherit: Inherit via back propagation
  LatchTime_SY : Constant  OutDataTypeStr=uint16  SampleTime=-1
  Memory : Memory  InheritSampleTime=on
  Relational Operator : RelationalOperator  Operator=<=  OutDataTypeStr=boolean  RndMeth=Nearest
  Saturation Dynamic : simulink/Discontinuities/Saturation Dynamic  OutMin=[]  OutMax=[]  OutDataTypeStr=Inherit: Same as second input  OutDataType=fixdt(1, 16)  OutScaling=2^-10  DoSatur=off
  Saturation2 : Saturate  UpperLimit=10000  LowerLimit=0  OutDataTypeStr=uint16
  Switch : Switch  Criteria=u2 > Threshold
  delta fall limit : Product  DisableCoverage=on  Inputs=**  OutDataTypeStr=Inherit: Inherit via back propagation  SaturateOnIntegerOverflow=on
  delta rise limit : Product  DisableCoverage=on  Inputs=**  OutDataTypeStr=Inherit: Inherit via back propagation  SaturateOnIntegerOverflow=on
  sample time : SampleTimeMath  DisableCoverage=on  TsampMathOp=Ts Only  weightValue=1
  Y : Outport
  wires:
  Delay Input2/1 -> Switch/3  "Y(k-1)"
  Relational Operator/1 -> Switch/2
  Constant/1 -> Add1/1
  LatchTime_SY/1 -> Relational Operator/2
  Saturation2/1 -> Memory/1
  Memory/1 -> Add1/2
  Add1/1 -> Saturation2/1, Relational Operator/1
  delta fall limit/1 -> Saturation Dynamic/3
  Difference Inputs1/1 -> Saturation Dynamic/2  "( U(k) - Y(k-1) )"
  Switch/1 -> Difference Inputs1/2, Difference Inputs2/2  "Y(k-1)"
  Saturation Dynamic/1 -> Difference Inputs2/1
  Difference Inputs2/1 -> Delay Input2/1, Y/1
  delta rise limit/1 -> Saturation Dynamic/1
  up/1 -> delta rise limit/1
  lo/1 -> delta fall limit/1
  sample time/1 -> delta rise limit/2, delta fall limit/2
  u/1 -> Difference Inputs1/1, Switch/1, sample time/1

== system D53_LKAS_JLU_20200909_1512/LL/LLOn/LKA/Lane Following (LF)/Preview Information Calculation (PIC) ==
  PIC_bsLKAInPInfo : Inport
  Add : Sum
  Add1 : Sum
  Add2 : Sum
  Bus Creator1 : BusCreator  Inputs=5
  Bus Selector1 : BusSelector  OutputSignals=Pr_bsPrInfo.bsPrDvtInfo.lPrvwDvtLft,Pr_bsPrInfo.bsPrDvtInfo.lPrvwDvtRgt,Pr_bsPrInfo.bsPrHdAgInfo.phiPrvwHdAgLft,Pr_bsPrInfo.bsPrHdAgInfo.phiPrvwHdAgRgt,Pr_bsPrInfo.bsPrCrvtInfo.crPrvwCrvtLft,Pr_bsPrInfo.bsPrCrvtInfo.crPrvwCrvtRgt,TTLC_bsTTLCInfo.vLft,TTLC_bsTTLCInfo.vRgt
  Gain : Gain  Gain=0.5
  Gain1 : Gain  Gain=0.5
  Gain2 : Gain  Gain=0.5
  PIC_bsPrvwInfo : Outport
  wires:
  Gain2/1 -> Bus Creator1/1  "PIC_lPrvwDvt"
  Bus Selector1/8 -> Bus Creator1/5  "<vRgt>"
  Bus Selector1/7 -> Bus Creator1/4  "<vLft>"
  Bus Selector1/5 -> Add2/1  "<crPrvwCrvtLft>"
  Bus Selector1/3 -> Add/1  "<phiPrvwHdAgLft>"
  Add/1 -> Gain/1
  Bus Selector1/6 -> Add2/2  "<crPrvwCrvtRgt>"
  Gain/1 -> Bus Creator1/2  "PIC_phiPrvwHdAg"
  Add1/1 -> Gain2/1
  Bus Selector1/4 -> Add/2  "<phiPrvwHdAgRgt>"
  Gain1/1 -> Bus Creator1/3  "PIC_crPrvwCrvt"
  Add2/1 -> Gain1/1
  Bus Selector1/2 -> Add1/2  "<lPrvwDvtRgt>"
  Bus Selector1/1 -> Add1/1  "<lPrvwDvtLft>"
  PIC_bsLKAInPInfo/1 -> Bus Selector1/1
  Bus Creator1/1 -> PIC_bsPrvwInfo/1

== system D53_LKAS_JLU_20200909_1512/LL/LLOn/LKA/Lane Following (LF)/Trajectory Following Control (TFC) ==
  TFC_bsPrvwInfo : Inport
  TFC_bsInInfoSyn : Inport  Port=2
  TFC_bsTFCClb : Inport  Port=3
  TFC_bsConstantClb : Inport  Port=4
  Bus Selector : BusSelector  OutputSignals=PIC_lPrvwDvt,PIC_phiPrvwHdAg,PIC_crPrvwCrvt
  Bus Selector1 : BusSelector  OutputSignals=LL_LFClb_TFC_tiKlatPrvwT_C,LL_LFClb_TFC_facmKlat_C,LL_LFClb_TFC_vGainLutVehSpdLwr_C,LL_LFClb_TFC_vGainLutVehSpdUpr_C,LL_LFClb_TFC_facmGainLutGain1_C,LL_LFClb_TFC_facmGainLutGain2_C,LL_LFClb_TFC_phiIntegCtlMaxSWA_C,LL_LFClb_TFC_facmIntegRatio,LL_LFClb_TFC_DiffCtrlRatio,LL_LFClb_TFC_DiffCtrlMaxSWA,LL_LFClb_TFC_DiffCtlBalance,LL_LFClb_TFC_FfCtlRatio_C
  Bus Selector2 : BusSelector  OutputSignals=LKA_WhlBaseL_C,LKA_StrRatio_C
  Bus Selector3 : BusSelector  OutputSignals=bsLaneInfo.bsL0Info,bsLaneInfo.bsR0Info,bsVehMovInfo.ESC_VehSpd
  Feedback Control (FbCtl) : Subsystem
  Feedforward Control (FfCtl) : Subsystem
  TFC_phiFfSWACmd : Outport
  TFC_phiPropSWACmd : Outport  Port=2
  TFC_phiIntegSWACmd : Outport  Port=3
  TFC_phiDiffSWACmd : Outport  Port=4
  wires:
  Bus Selector1/11 -> Feedback Control (FbCtl)/17(FbCtl_DiffCtlBalance)  "<LL_LFClb_TFC_DiffCtlBalance>"
  Bus Selector1/9 -> Feedback Control (FbCtl)/15(FbCtl_DiffCtlRatioIn)  "<LL_LFClb_TFC_DiffCtrlRatio>"
  Bus Selector1/10 -> Feedback Control (FbCtl)/16(FbCtl_DiffCtlMaxSWA)  "<LL_LFClb_TFC_DiffCtrlMaxSWA>"
  Feedback Control (FbCtl)/2(FbCtl_phiFbIntegCtlSWA) -> TFC_phiIntegSWACmd/1
  Bus Selector1/8 -> Feedback Control (FbCtl)/14(FbCtl_facmIntegRatio)  "<LL_LFClb_TFC_facmIntegRatio>"
  Bus Selector1/7 -> Feedback Control (FbCtl)/13(FbCtl_phiIntegCtlMaxSWA_C)  "<LL_LFClb_TFC_phiIntegCtlMaxSWA_C>"
  Bus Selector1/12 -> Feedforward Control (FfCtl)/1(FfCtl_FfCtlRatio_C)  "<LL_LFClb_TFC_FfCtlRatio_C>"
  TFC_bsConstantClb/1 -> Bus Selector2/1
  Bus Selector2/2 -> Feedforward Control (FfCtl)/5(FfCtl_rTraRatio_C)  "<LKA_StrRatio_C>"
  Bus Selector2/1 -> Feedforward Control (FfCtl)/4(FfCtl_lWhlBase_SY)  "<LKA_WhlBaseL_C>"
  Bus Selector1/6 -> Feedback Control (FbCtl)/12(FbCtl_facmGainLimUpr_C)  "<LL_LFClb_TFC_facmGainLutGain2_C>"
  Bus Selector1/5 -> Feedback Control (FbCtl)/11(FbCtl_facmGainLimLwr_C)  "<LL_LFClb_TFC_facmGainLutGain1_C>"
  Bus Selector1/4 -> Feedback Control (FbCtl)/10(FbCtl_vVehSpdLimUpr_C)  "<LL_LFClb_TFC_vGainLutVehSpdUpr_C>"
  Bus Selector1/3 -> Feedback Control (FbCtl)/9(FbCtl_vVehSpdLimLwr_C)  "<LL_LFClb_TFC_vGainLutVehSpdLwr_C>"
  Bus Selector3/3 -> Feedforward Control (FfCtl)/2(FfCtl_vVehSpd), Feedback Control (FbCtl)/3(FbCtl_vVehSpd)  "<ESC_VehSpd>"
  Bus Selector1/2 -> Feedback Control (FbCtl)/8(FbCtl_facmKlat_C)  "<LL_LFClb_TFC_facmKlat_C>"
  Bus Selector1/1 -> Feedback Control (FbCtl)/7(FbCtl_tiKlatPrvwT_C)  "<LL_LFClb_TFC_tiKlatPrvwT_C>"
  TFC_bsTFCClb/1 -> Bus Selector1/1
  Bus Selector/2 -> Feedback Control (FbCtl)/5(FbCtl_phiPrvwHdAg)  "<PIC_phiPrvwHdAg>"
  Bus Selector/1 -> Feedback Control (FbCtl)/4(FbCtl_lPrvwDvt)  "<PIC_lPrvwDvt>"
  TFC_bsPrvwInfo/1 -> Bus Selector/1  "bsPrvwInfo"
  Feedback Control (FbCtl)/1(FbCtl_phiFbPropCtlSWA) -> TFC_phiPropSWACmd/1
  Feedforward Control (FfCtl)/1(FfCtl_phiFfSWA) -> TFC_phiFfSWACmd/1  "phiFfSWA"
  Bus Selector/3 -> Feedback Control (FbCtl)/6(FbCtl_crPrvwCrvt), Feedforward Control (FfCtl)/3(FfCtl_crPrvwCrvt)  "<PIC_crPrvwCrvt>"
  TFC_bsInInfoSyn/1 -> Bus Selector3/1
  Bus Selector3/1 -> Feedback Control (FbCtl)/1(FbCtl_bsL0Info)  "<bsL0Info>"
  Bus Selector3/2 -> Feedback Control (FbCtl)/2(FbCtl_bsR0Info)  "<bsR0Info>"
  Feedback Control (FbCtl)/3(FbCtl_phiFbDiffCtlSWA) -> TFC_phiDiffSWACmd/1

== system D53_LKAS_JLU_20200909_1512/LL/LLOn/LKA/Plan To LaneFollowing (PTLF)/InsideJudge ==
  Flg : Inport
  Crvt : Inport  Port=2
  Compare To Constant : simulink/Logic and Bit Operations/Compare To Constant  relop===  const=1  OutDataTypeStr=boolean
  Compare To Constant1 : simulink/Logic and Bit Operations/Compare To Constant  relop===  const=2  OutDataTypeStr=boolean
  Constant : Constant  Value=0.001  OutDataTypeStr=single
  Constant3 : Constant  Value=-0.001  OutDataTypeStr=single
  Logical Operator : Logic  AllPortsSameDT=off  OutDataTypeStr=boolean
  Logical Operator1 : Logic  AllPortsSameDT=off  OutDataTypeStr=boolean
  Logical Operator2 : Logic  Operator=OR  AllPortsSameDT=off  OutDataTypeStr=boolean
  Relational Operator : RelationalOperator  OutDataTypeStr=boolean  RndMeth=Simplest
  Relational Operator1 : RelationalOperator  Operator=<=  OutDataTypeStr=boolean  RndMeth=Simplest
  Out1 : Outport
  wires:
  Crvt/1 -> Relational Operator/1, Relational Operator1/1
  Logical Operator2/1 -> Out1/1
  Constant3/1 -> Relational Operator1/2
  Relational Operator1/1 -> Logical Operator1/2  "LeftCrvt"
  Constant/1 -> Relational Operator/2
  Compare To Constant1/1 -> Logical Operator/1  "RightActive"
  Relational Operator/1 -> Logical Operator/2  "RightCrvt"
  Flg/1 -> Compare To Constant/1, Compare To Constant1/1
  Logical Operator/1 -> Logical Operator2/2
  Logical Operator1/1 -> Logical Operator2/1
  Compare To Constant/1 -> Logical Operator1/1  "LeftActive"

== system D53_LKAS_JLU_20200909_1512/LL/LLOn/LKA/Plan To LaneFollowing (PTLF)/InsideJudge1 ==
  Flg : Inport
  HdAgLft : Inport  Port=2
  HdAgRgt : Inport  Port=3
  T1 : Inport  Port=4
  Plan : Inport  Port=5
  Time : Inport  Port=6
  If : If  IfExpression=u1 == 1  ElseIfExpressions=u1 == 2
  If Action Subsystem : Subsystem  TreatAsAtomicUnit=on
  If Action Subsystem1 : Subsystem  TreatAsAtomicUnit=on
  If Action Subsystem2 : Subsystem  TreatAsAtomicUnit=on
  Merge : Merge  Inputs=3  InitialOutput=1
  Merge1 : Merge  Inputs=3  InitialOutput=0
  T1_1 : Outport
  Plan_1 : Outport  Port=2
  wires:
  Time/1 -> If Action Subsystem/4(Time), If Action Subsystem1/4(Time)
  Merge1/1 -> Plan_1/1
  Merge/1 -> T1_1/1
  HdAgRgt/1 -> If Action Subsystem1/3(HdAgRgt)
  Plan/1 -> If Action Subsystem2/2(Plan), If Action Subsystem1/2(Plan), If Action Subsystem/2(Plan)
  T1/1 -> If Action Subsystem2/1(T1), If Action Subsystem1/1(T1), If Action Subsystem/1(T1)
  If Action Subsystem2/2(Plan_1) -> Merge1/3
  If Action Subsystem1/2(Plan_1) -> Merge1/2
  If Action Subsystem/2(Plan_1) -> Merge1/1
  If Action Subsystem2/1(T1_1) -> Merge/3
  If Action Subsystem1/1(T1_1) -> Merge/2
  If Action Subsystem/1(T1_1) -> Merge/1
  HdAgLft/1 -> If Action Subsystem/3(HdAgLft)
  If/3 -> If Action Subsystem2/Action
  If/2 -> If Action Subsystem1/Action
  If/1 -> If Action Subsystem/Action
  Flg/1 -> If/1

== system D53_LKAS_JLU_20200909_1512/LL/LLOn/LKA/Plan To LaneFollowing (PTLF)/LowPass ==
  T : Inport
  u : Inport  Port=2
  dT : Inport  Port=3
  Add : Sum  Inputs=+-
  Add1 : Sum
  Add2 : Sum  OutDataTypeStr=single
  Divide : Product  Inputs=*/
  Divide1 : Product  Inputs=**
  Memory3 : Memory  InheritSampleTime=on
  SWACmdSyn_tiSmplT_C4 : Constant  OutDataTypeStr=single
  Saturation : Saturate  UpperLimit=50  LowerLimit=0
  Switch : Switch  Criteria=u2 > Threshold  Threshold=30
  Unit Delay : UnitDelay  SampleTime=-1
  y : Outport
  wires:
  T/1 -> Divide/2
  dT/1 -> Divide/1
  u/1 -> Switch/3, Add/1
  Divide/1 -> Divide1/1
  Add/1 -> Divide1/2
  Divide1/1 -> Add1/1
  Unit Delay/1 -> Add/2, Add1/2
  Add1/1 -> Switch/1
  SWACmdSyn_tiSmplT_C4/1 -> Add2/1
  Add2/1 -> Saturation/1
  Saturation/1 -> Switch/2, Memory3/1
  Memory3/1 -> Add2/2
  Switch/1 -> y/1, Unit Delay/1

== system D53_LKAS_JLU_20200909_1512/LL/LLOn/LKA/Plan To LaneFollowing (PTLF)/TickTime (TTime) ==
  Add2 : Sum  OutDataTypeStr=single
  Memory3 : Memory  InheritSampleTime=on
  Saturation : Saturate  UpperLimit=50  LowerLimit=0
  Out1 : Outport
  wires:
  [LKA_SampleTime] -> Add2/1
  Saturation/1 -> Memory3/1, Out1/1
  Memory3/1 -> Add2/2
  Add2/1 -> Saturation/1

== system D53_LKAS_JLU_20200909_1512/LL/LLOn/LKA/Plan To LaneFollowing (PTLF)/TimeGain ==
  Time : Inport
  T1 : Inport  Port=2
  TFC : Inport  Port=3
  Add1 : Sum
  Add2 : Sum  Inputs=+-
  Add3 : Sum  Inputs=-+
  Constant1 : Constant  Value=0  OutDataTypeStr=single
  Constant4 : Constant  OutDataTypeStr=single
  Divide : Product  Inputs=*/
  Divide8 : Product  Inputs=**
  Saturation4 : Saturate  UpperLimit=1  LowerLimit=0
  Out1 : Outport
  wires:
  Add3/1 -> Divide8/1
  Constant4/1 -> Add3/2
  Add2/1 -> Divide/1
  Divide/1 -> Saturation4/1
  Time/1 -> Add2/1
  T1/1 -> Add2/2
  TFC/1 -> Divide/2
  Add1/1 -> Out1/1
  Divide8/1 -> Add1/2
  Constant1/1 -> Add3/1, Add1/1
  Saturation4/1 -> Divide8/2

== system D53_LKAS_JLU_20200909_1512/LL/LLOn/LKA Input Processing (LKAInP)/Predicted Deviation Calculation (PrDvt)/Lane Information Selection (LaneInfoSel) ==
  LaneInfoSel_stLKAActvFlg : Inport
  LaneInfoSel_facmLftLane : Inport  Port=2
  LaneInfoSel_facmRgtLane : Inport  Port=3
  If : If  IfExpression=u1==1  ElseIfExpressions=u1==2
  If Action Subsystem1 : Subsystem  TreatAsAtomicUnit=on
  If Action Subsystem2 : Subsystem  TreatAsAtomicUnit=on
  If Action Subsystem3 : Subsystem  TreatAsAtomicUnit=on
  Merge : Merge  Inputs=3
  LaneInfoSel_facmActvLane : Outport
  wires:
  LaneInfoSel_facmRgtLane/1 -> If Action Subsystem1/1(In1), If Action Subsystem3/2(In2)
  LaneInfoSel_facmLftLane/1 -> If Action Subsystem2/1(In1), If Action Subsystem3/1(In1)
  LaneInfoSel_stLKAActvFlg/1 -> If/1
  If/1 -> If Action Subsystem2/Action
  If Action Subsystem2/1(Out1) -> Merge/1
  Merge/1 -> LaneInfoSel_facmActvLane/1
  If/2 -> If Action Subsystem1/Action
  If Action Subsystem1/1(Out1) -> Merge/2
  If Action Subsystem3/1(Out1) -> Merge/3
  If/3 -> If Action Subsystem3/Action

== system D53_LKAS_JLU_20200909_1512/LL/LLOn/LKA Input Processing (LKAInP)/Predicted Deviation Calculation (PrDvt)/Lane Information Selection (LaneInfoSel)1 ==
  LaneInfoSel_stLKAActvFlg : Inport
  LaneInfoSel_facmLftLane : Inport  Port=2
  LaneInfoSel_facmRgtLane : Inport  Port=3
  If : If  IfExpression=u1==1  ElseIfExpressions=u1==2
  If Action Subsystem1 : Subsystem  TreatAsAtomicUnit=on
  If Action Subsystem2 : Subsystem  TreatAsAtomicUnit=on
  If Action Subsystem3 : Subsystem  TreatAsAtomicUnit=on
  Merge : Merge  Inputs=3
  LaneInfoSel_facmActvLane : Outport
  wires:
  If/3 -> If Action Subsystem3/Action
  If Action Subsystem3/1(Out1) -> Merge/3
  If Action Subsystem1/1(Out1) -> Merge/2
  If/2 -> If Action Subsystem1/Action
  Merge/1 -> LaneInfoSel_facmActvLane/1
  If Action Subsystem2/1(Out1) -> Merge/1
  If/1 -> If Action Subsystem2/Action
  LaneInfoSel_stLKAActvFlg/1 -> If/1
  LaneInfoSel_facmLftLane/1 -> If Action Subsystem3/1(In1), If Action Subsystem2/1(In1)
  LaneInfoSel_facmRgtLane/1 -> If Action Subsystem3/2(In2), If Action Subsystem1/1(In1)

== system D53_LKAS_JLU_20200909_1512/LL/LLOn/LKA Input Processing (LKAInP)/Predicted Deviation Calculation (PrDvt)/Left Front Conner Deviation Calculation (LFCDvtCalc) ==
  PrdcDvt_bsPrHdAgInfo : Inport
  LFCDvtCalc_lDvt : Inport  Port=2
  LFCDvtCalc_lDvtComp_C : Inport  Port=3
  Add : Sum  Inputs=+-  OutDataTypeStr=single
  Add1 : Sum  OutDataTypeStr=single
  Add5 : Sum  OutDataTypeStr=single
  Bus Selector : BusSelector  OutputSignals=LKA_Veh2CamW_C,LKA_Veh2CamL_C
  Bus Selector2 : BusSelector  OutputSignals=phiHdAgLft
  Cos2 : Trigonometry  Operator=cos
  Divide : Product  Inputs=**
  Divide1 : Product  Inputs=**
  Gain1 : Gain  Gain=-1  OutDataTypeStr=single
  Sin : Trigonometry
  DvtCalc_lLftDvt : Outport
  wires:
  Add5/1 -> Gain1/1
  Add1/1 -> Divide/1
  Divide1/1 -> Add5/2
  Divide/1 -> Add5/1
  Sin/1 -> Divide1/2
  Cos2/1 -> Divide/2
  Gain1/1 -> DvtCalc_lLftDvt/1
  Bus Selector2/1 -> Cos2/1, Sin/1  "<phiHdAgLft>"
  Bus Selector/2 -> Divide1/1  "<LKA_Veh2CamL_C>"
  PrdcDvt_bsPrHdAgInfo/1 -> Bus Selector2/1
  [LLClb_bsConstantClb] -> Bus Selector/1
  Bus Selector/1 -> Add1/2  "<LKA_Veh2CamW_C>"
  Add/1 -> Add1/1
  LFCDvtCalc_lDvtComp_C/1 -> Add/2
  LFCDvtCalc_lDvt/1 -> Add/1

== system D53_LKAS_JLU_20200909_1512/LL/LLOn/LKA Input Processing (LKAInP)/Predicted Deviation Calculation (PrDvt)/Predicted Deviation Correction (PrdcDvtCor) ==
  PrdcDvtCor_bsPrdcHdAgInfo : Inport
  PrdcDvtCor_lPrvwDstZ : Inport  Port=2
  Bus Selector : BusSelector  OutputSignals=phiPrdcHdAgComp
  Divide2 : Product  Inputs=**  OutDataTypeStr=single
  PrdcDvtCor_lPrdcDvtCor : Outport
  wires:
  Divide2/1 -> PrdcDvtCor_lPrdcDvtCor/1
  PrdcDvtCor_lPrvwDstZ/1 -> Divide2/1
  PrdcDvtCor_bsPrdcHdAgInfo/1 -> Bus Selector/1
  Bus Selector/1 -> Divide2/2  "<phiPrdcHdAgComp>"

== system D53_LKAS_JLU_20200909_1512/LL/LLOn/LKA Input Processing (LKAInP)/Predicted Deviation Calculation (PrDvt)/Predicted Deviation of Left Lane Line (PrdcDvtLft) ==
  PrdcDvtLft_bsL0Info : Inport
  PrdcDvtLft_lPrvwDstZ : Inport  Port=2
  Add : Sum  Inputs=++++  AccumDataTypeStr=single
  Bus Selector : BusSelector  OutputSignals=L0_C0,L0_C1,L0_C2,L0_C3
  Product : Product  OutDataTypeStr=single  RndMeth=Zero
  Product3 : Product  OutDataTypeStr=single  RndMeth=Zero
  Product4 : Product  OutDataTypeStr=single  RndMeth=Zero
  Z*Z : Product  OutDataTypeStr=single  RndMeth=Zero
  Z*Z*Z : Product  OutDataTypeStr=single  RndMeth=Zero
  PrdcDvtLft_lPrdcDvtLft : Outport
  wires:
  Add/1 -> PrdcDvtLft_lPrdcDvtLft/1
  PrdcDvtLft_bsL0Info/1 -> Bus Selector/1
  PrdcDvtLft_lPrvwDstZ/1 -> Z*Z*Z/1, Z*Z/1, Product/2, Z*Z/2
  Bus Selector/2 -> Product/1  "<L0_C1>"
  Product/1 -> Add/2
  Bus Selector/1 -> Add/1  "<L0_C0>"
  Product3/1 -> Add/3
  Bus Selector/3 -> Product3/1  "<L0_C2>"
  Bus Selector/4 -> Product4/1  "<L0_C3>"
  Product4/1 -> Add/4
  Z*Z*Z/1 -> Product4/2
  Z*Z/1 -> Product3/2, Z*Z*Z/2

== system D53_LKAS_JLU_20200909_1512/LL/LLOn/LKA Input Processing (LKAInP)/Predicted Deviation Calculation (PrDvt)/Predicted Deviation of Left Line (PrdcDvtLft) ==
  PrdcDvtLft_bsPrdcHdAgInfo : Inport
  PrdcDvtLft_lPrdcDvtCor : Inport  Port=2
  PrdcDvtLft_lPrdcDvtLft : Inport  Port=3
  PrdcDvtLft_lDvtComp_C : Inport  Port=4
  " " : MATLAB Function  TreatAsAtomicUnit=on
  Add : Sum  Inputs=+-  AccumDataTypeStr=single  OutDataTypeStr=single
  Add1 : Sum  AccumDataTypeStr=single  OutDataTypeStr=single
  Add3 : Sum  AccumDataTypeStr=single  OutDataTypeStr=single
  Bus Selector : BusSelector  OutputSignals=phiPrvwTTLCHdAgLft,phiPrdcTTLCHdAg
  Bus Selector1 : BusSelector  OutputSignals=LKA_Veh2CamW_C,LKA_Veh2CamL_C
  Fcn3 : Fcn  Commented=on  Expr=u(2)*cos(u(1))+u(3)*sin(u(1))
  MATLAB Function : MATLAB Function  TreatAsAtomicUnit=on
  PrdcDvtLft_lDvtLft : Outport
  wires:
  [LLClb_bsConstantClb] -> Bus Selector1/1
  " "/1(y) -> Add1/2
  PrdcDvtLft_lPrdcDvtLft/1 -> Add/1
  PrdcDvtLft_lDvtComp_C/1 -> Add/2
  Add/1 -> MATLAB Function/1(u1)
  MATLAB Function/1(y) -> Add1/1
  PrdcDvtLft_lPrdcDvtCor/1 -> Add3/2  "PrdcDvtLft"
  Bus Selector1/2 -> " "/3(u3)  "<LKA_Veh2CamL_C>"
  Add1/1 -> Add3/1  "PrvwDvtLft"
  Add3/1 -> PrdcDvtLft_lDvtLft/1
  PrdcDvtLft_bsPrdcHdAgInfo/1 -> Bus Selector/1
  Bus Selector/1 -> MATLAB Function/2(u2)  "<phiPrvwTTLCHdAgLft>"
  Bus Selector/2 -> " "/1(u1)  "<phiPrdcTTLCHdAg>"
  Bus Selector1/1 -> " "/2(u2)  "<LKA_Veh2CamW_C>"
